simulink model "MDFM2"  (R2023a)
settings: Solver=FixedStepDiscrete  StartTime=0.0  StopTime=10.0  FixedStep=0.0001  RelTol=1e-3  EnableMultiTasking=on
undefined symbols (not defined in the file or in its folder): GLBCal_GLBCal_Kf_DCLinkOverVolErrThd_V, GLBCal_GLBCal_Kf_DCLinkUnderVolErrThd_V, KfMDFM_DCLinkOverVolWarnThd_V, KfMDFM_DCLinkUnderVolWarnThd_V, KfMDFM_OverVolPowerOutoutSetPoint_V, KfMDFM_OverVolPowerOutputFactor_NULL, KfMDFM_UnderVolPowerOutoutSetPoint_V, KfMDFM_UnderVolPowerOutputFactor_NULL, KuMDFM_DCLinkOVECntDownLimit_NULL, KuMDFM_DCLinkOVECntDownRate_NULL, KuMDFM_DCLinkOVECntUpLimit_NULL, KuMDFM_DCLinkOVECntUpRate_NULL, KuMDFM_DCLinkOVWCntDownLimit_NULL, KuMDFM_DCLinkOVWCntDownRate_NULL, KuMDFM_DCLinkOVWCntUpLimit_NULL, KuMDFM_DCLinkOVWCntUpRate_NULL, KuMDFM_DCLinkUVECntDownLimit_NULL, KuMDFM_DCLinkUVECntDownRate_NULL, KuMDFM_DCLinkUVECntUpLimit_NULL, KuMDFM_DCLinkUVECntUpRate_NULL, KuMDFM_DCLinkUVWCntDownLimit_NULL, KuMDFM_DCLinkUVWCntDownRate_NULL, KuMDFM_DCLinkUVWCntUpLimit_NULL, KuMDFM_DCLinkUVWCntUpRate_NULL, MDPM_MCUStatus, MDSM_MCUStatus
libraries: simulink x8, PMSM_Library x5
settings Model: DataDictionary=PMSM_Merge.sldd  EnableAccessToBaseWorkspace=off  Creator=yuliang  LastModifiedBy=洲
settings SolverCC: AlgebraicLoopSolver=TrustRegion
settings DataIOCC: LimitDataPoints=on  SaveFormat=StructureWithTime  ReturnWorkspaceOutputs=off
settings OptimizationCC: DefaultParameterBehavior=Inlined  DefaultUnderspecifiedDataType=single  EnhancedBackFolding=on  PassReuseOutputArgsAs=Individual arguments  ZeroExternalMemoryAtStartup=off  ZeroInternalMemoryAtStartup=off  OptimizeBlockOrder=speed  DifferentSizesBufferReuse=on  OptimizationCustomize=off  EfficientTunableParamExpr=on
settings DebuggingCC: ParameterTunabilityLossMsg=error  UnconnectedInputMsg=warning  UnconnectedOutputMsg=warning  UnconnectedLineMsg=warning  AllowSymbolicDim=off  SFUnexpectedBacktrackingDiag=warning  SFNoUnconditionalDefaultTransitionDiag=warning  SFExecutionAtInitializationDiag=none  ArithmeticOperatorsInVariantConditions=warning
settings HardwareCC: ProdBitPerPointer=32  ProdBitPerSizeT=32  ProdBitPerPtrDiffT=32  ProdLargestAtomicFloat=None  ProdWordSize=32  ProdHWDeviceType=Infineon->TriCore
settings ModelReferenceCC: EnableRefExpFcnMdlSchedulingChecks=on  ModelReferenceNumInstancesAllowed=Single  PropagateSignalLabelsOutOfModel=off
settings SFSimCC: SimUseLocalCustomCode=off  MATLABDynamicMemAlloc=off  CustomCodeUndefinedFunction=UseInterfaceOnly
settings RTWCC: Description=AUTOSAR  SystemTargetFile=autosar.tlc  GenCodeOnly=on  TemplateMakefile=ert_default_tmf  GenerateReport=on  RTWUseLocalCustomCode=off  IncludeHyperlinkInReport=on  LaunchReport=on  GenerateTraceInfo=on  GenerateTraceReport=on  GenerateTraceReportSl=on  GenerateTraceReportSf=on  GenerateTraceReportEml=on  DLArmComputeVersion=19.05
settings CodeAppCC: ForceParamTrailComments=on  IgnoreCustomStorageClasses=off  OperatorAnnotations=on  SimulinkDataObjDesc=on  SFDataObjDesc=on  InsertBlockDesc=on
settings STFCustomTargetCC: TargetLangStandard=C89/C90 (ANSI)  MultiwordLength=256  ParMdlRefBuildCompliant=on  CompOptLevelCompliant=on  ConcurrentExecutionCompliant=off  IncludeMdlTerminateFcn=off  CombineOutputUpdateFcns=on  SuppressErrorStatus=on  ERTCustomFileBanners=on  SupportNonFinite=off  SupportComplex=off  SupportContinuousTime=off  SupportNonInlinedSFcns=off  RemoveResetFunc=on  MATLABClassNameForMDSCustomization=Simulink.SoftwareTarget.ERTCustomization  AutosarCompliant=on  GRTInterface=off  LookupTableObjectStructAxisOrder=2,1,3,4,...  LUTObjectStructOrderEvenSpacing=Size,Table,Breakpoints  SystemTargetFile=autosar.tlc
settings ERTTargetCC: ConcurrentExecutionCompliant=off  IncludeMdlTerminateFcn=off  SuppressErrorStatus=on  SupportNonFinite=off  SupportComplex=off  ModelStepFunctionPrototypeControlCompliant=off  CPPClassGenCompliant=off  AutosarCompliant=on  LookupTableObjectStructAxisOrder=2,1,3,4,...  LUTObjectStructOrderEvenSpacing=Size,Table,Breakpoints  InlinedParameterPlacement=NonHierarchical  ERTCustomFileTemplate=example_file_process.tlc
settings ConfigComp: CovMetricSettings=dw  CovSaveCumulativeToWorkspaceVar=on  CovSaveSingleToWorkspaceVar=on  CovExternalEMLEnable=off

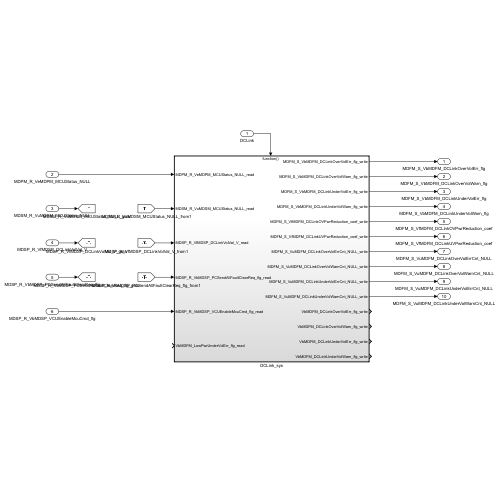
[thumbnail: Simulink's stored preview of the top-level diagram]
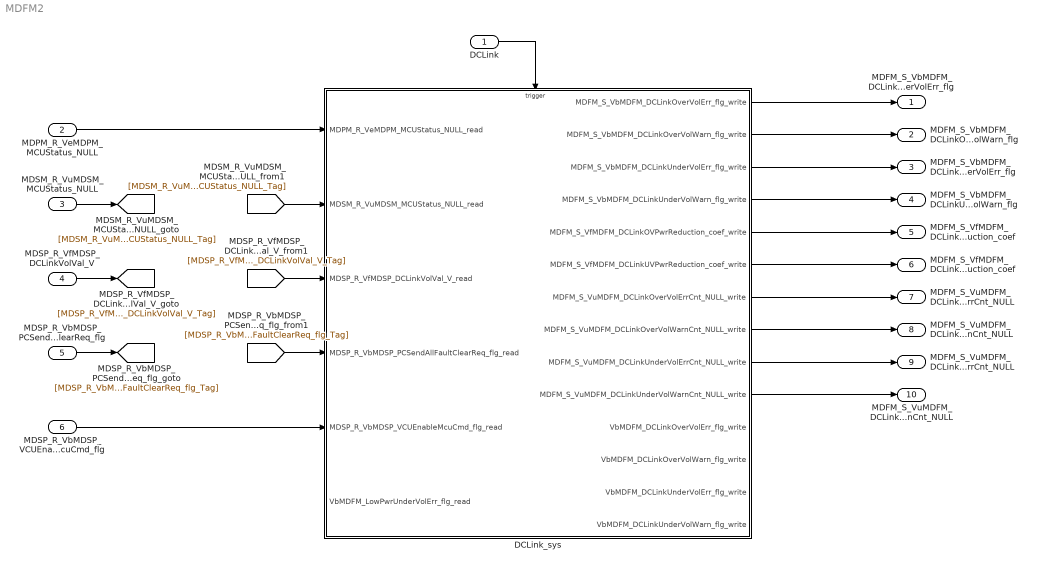
== system MDFM2 ==
  DCLink : Inport  SampleTime=0.005  OutputFunctionCall=on
  MDPM_R_VeMDPM_MCUStatus_NULL : Inport  Port=2  OutDataTypeStr=uint8  PortDimensions=1
  MDSM_R_VuMDSM_MCUStatus_NULL : Inport  Port=3  OutDataTypeStr=uint16  PortDimensions=1
  MDSP_R_VfMDSP_DCLinkVolVal_V : Inport  Port=4  OutDataTypeStr=single  PortDimensions=1
  MDSP_R_VbMDSP_PCSendAllFaultClearReq_flg : Inport  Port=5  OutDataTypeStr=boolean  PortDimensions=1
  MDSP_R_VbMDSP_VCUEnableMcuCmd_flg : Inport  Port=6  OutDataTypeStr=boolean  PortDimensions=1
  DCLink_sys : Subsystem
  MDFM_S_VbMDFM_DCLinkOverVolErr_flg : Outport  OutDataTypeStr=boolean  PortDimensions=1
  MDFM_S_VbMDFM_DCLinkOverVolWarn_flg : Outport  Port=2  OutDataTypeStr=boolean  PortDimensions=1
  MDFM_S_VbMDFM_DCLinkUnderVolErr_flg : Outport  Port=3  OutDataTypeStr=boolean  PortDimensions=1
  MDFM_S_VbMDFM_DCLinkUnderVolWarn_flg : Outport  Port=4  OutDataTypeStr=boolean  PortDimensions=1
  MDFM_S_VfMDFM_DCLinkOVPwrReduction_coef : Outport  Port=5  OutDataTypeStr=single  PortDimensions=1
  MDFM_S_VfMDFM_DCLinkUVPwrReduction_coef : Outport  Port=6  OutDataTypeStr=single  PortDimensions=1
  MDFM_S_VuMDFM_DCLinkOverVolErrCnt_NULL : Outport  Port=7  OutDataTypeStr=uint16  PortDimensions=1
  MDFM_S_VuMDFM_DCLinkOverVolWarnCnt_NULL : Outport  Port=8  OutDataTypeStr=uint16  PortDimensions=1
  MDFM_S_VuMDFM_DCLinkUnderVolErrCnt_NULL : Outport  Port=9  OutDataTypeStr=uint16  PortDimensions=1
  MDFM_S_VuMDFM_DCLinkUnderVolWarnCnt_NULL : Outport  Port=10  OutDataTypeStr=uint16  PortDimensions=1
  wires:
  DCLink/1 -> DCLink_sys/Trigger
  MDPM_R_VeMDPM_MCUStatus_NULL/1 -> DCLink_sys/1(MDPM_R_VeMDPM_MCUStatus_NULL_read)
  MDSM_R_VuMDSM_MCUStatus_NULL/1 -> [MDSM_R_VuMDSM_MCUStatus_NULL_Tag]
  [MDSM_R_VuMDSM_MCUStatus_NULL_Tag] -> DCLink_sys/2(MDSM_R_VuMDSM_MCUStatus_NULL_read)
  MDSP_R_VfMDSP_DCLinkVolVal_V/1 -> [MDSP_R_VfMDSP_DCLinkVolVal_V_Tag]
  [MDSP_R_VfMDSP_DCLinkVolVal_V_Tag] -> DCLink_sys/3(MDSP_R_VfMDSP_DCLinkVolVal_V_read)
  MDSP_R_VbMDSP_PCSendAllFaultClearReq_flg/1 -> [MDSP_R_VbMDSP_PCSendAllFaultClearReq_flg_Tag]
  [MDSP_R_VbMDSP_PCSendAllFaultClearReq_flg_Tag] -> DCLink_sys/4(MDSP_R_VbMDSP_PCSendAllFaultClearReq_flg_read)
  MDSP_R_VbMDSP_VCUEnableMcuCmd_flg/1 -> DCLink_sys/5(MDSP_R_VbMDSP_VCUEnableMcuCmd_flg_read)
  DCLink_sys/1(MDFM_S_VbMDFM_DCLinkOverVolErr_flg_write) -> MDFM_S_VbMDFM_DCLinkOverVolErr_flg/1
  DCLink_sys/2(MDFM_S_VbMDFM_DCLinkOverVolWarn_flg_write) -> MDFM_S_VbMDFM_DCLinkOverVolWarn_flg/1
  DCLink_sys/3(MDFM_S_VbMDFM_DCLinkUnderVolErr_flg_write) -> MDFM_S_VbMDFM_DCLinkUnderVolErr_flg/1
  DCLink_sys/4(MDFM_S_VbMDFM_DCLinkUnderVolWarn_flg_write) -> MDFM_S_VbMDFM_DCLinkUnderVolWarn_flg/1
  DCLink_sys/5(MDFM_S_VfMDFM_DCLinkOVPwrReduction_coef_write) -> MDFM_S_VfMDFM_DCLinkOVPwrReduction_coef/1
  DCLink_sys/6(MDFM_S_VfMDFM_DCLinkUVPwrReduction_coef_write) -> MDFM_S_VfMDFM_DCLinkUVPwrReduction_coef/1
  DCLink_sys/7(MDFM_S_VuMDFM_DCLinkOverVolErrCnt_NULL_write) -> MDFM_S_VuMDFM_DCLinkOverVolErrCnt_NULL/1
  DCLink_sys/8(MDFM_S_VuMDFM_DCLinkOverVolWarnCnt_NULL_write) -> MDFM_S_VuMDFM_DCLinkOverVolWarnCnt_NULL/1
  DCLink_sys/9(MDFM_S_VuMDFM_DCLinkUnderVolErrCnt_NULL_write) -> MDFM_S_VuMDFM_DCLinkUnderVolErrCnt_NULL/1
  DCLink_sys/10(MDFM_S_VuMDFM_DCLinkUnderVolWarnCnt_NULL_write) -> MDFM_S_VuMDFM_DCLinkUnderVolWarnCnt_NULL/1

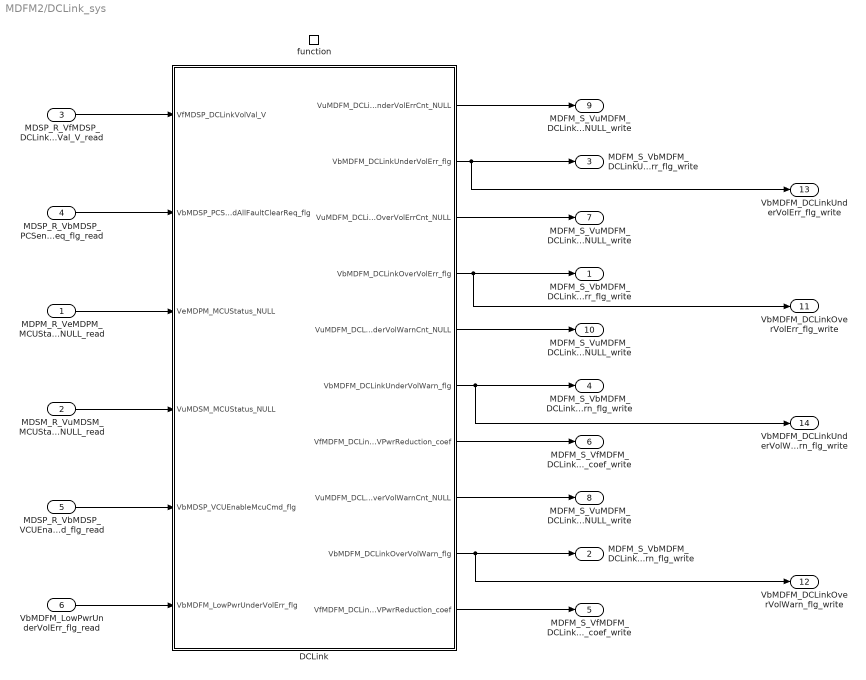
== system MDFM2/DCLink_sys ==
  MDPM_R_VeMDPM_MCUStatus_NULL_read : Inport
  MDSM_R_VuMDSM_MCUStatus_NULL_read : Inport  Port=2
  MDSP_R_VfMDSP_DCLinkVolVal_V_read : Inport  Port=3
  MDSP_R_VbMDSP_PCSendAllFaultClearReq_flg_read : Inport  Port=4
  MDSP_R_VbMDSP_VCUEnableMcuCmd_flg_read : Inport  Port=5
  VbMDFM_LowPwrUnderVolErr_flg_read : Inport  Port=6
  function : TriggerPort  TriggerType=function-call  VariantControl=Variant  SampleTimeType=periodic  SampleTime=-1
  DCLink : Subsystem
  MDFM_S_VbMDFM_DCLinkOverVolErr_flg_write : Outport
  MDFM_S_VbMDFM_DCLinkOverVolWarn_flg_write : Outport  Port=2
  MDFM_S_VbMDFM_DCLinkUnderVolErr_flg_write : Outport  Port=3
  MDFM_S_VbMDFM_DCLinkUnderVolWarn_flg_write : Outport  Port=4
  MDFM_S_VfMDFM_DCLinkOVPwrReduction_coef_write : Outport  Port=5
  MDFM_S_VfMDFM_DCLinkUVPwrReduction_coef_write : Outport  Port=6
  MDFM_S_VuMDFM_DCLinkOverVolErrCnt_NULL_write : Outport  Port=7
  MDFM_S_VuMDFM_DCLinkOverVolWarnCnt_NULL_write : Outport  Port=8
  MDFM_S_VuMDFM_DCLinkUnderVolErrCnt_NULL_write : Outport  Port=9
  MDFM_S_VuMDFM_DCLinkUnderVolWarnCnt_NULL_write : Outport  Port=10
  VbMDFM_DCLinkOverVolErr_flg_write : Outport  Port=11  OutDataTypeStr=boolean  PortDimensions=1
  VbMDFM_DCLinkOverVolWarn_flg_write : Outport  Port=12  OutDataTypeStr=boolean  PortDimensions=1
  VbMDFM_DCLinkUnderVolErr_flg_write : Outport  Port=13  OutDataTypeStr=boolean  PortDimensions=1
  VbMDFM_DCLinkUnderVolWarn_flg_write : Outport  Port=14  OutDataTypeStr=boolean  PortDimensions=1
  wires:
  MDPM_R_VeMDPM_MCUStatus_NULL_read/1 -> DCLink/3(VeMDPM_MCUStatus_NULL)
  MDSM_R_VuMDSM_MCUStatus_NULL_read/1 -> DCLink/4(VuMDSM_MCUStatus_NULL)
  MDSP_R_VfMDSP_DCLinkVolVal_V_read/1 -> DCLink/1(VfMDSP_DCLinkVolVal_V)
  MDSP_R_VbMDSP_PCSendAllFaultClearReq_flg_read/1 -> DCLink/2(VbMDSP_PCSendAllFaultClearReq_flg)
  MDSP_R_VbMDSP_VCUEnableMcuCmd_flg_read/1 -> DCLink/5(VbMDSP_VCUEnableMcuCmd_flg)
  VbMDFM_LowPwrUnderVolErr_flg_read/1 -> DCLink/6(VbMDFM_LowPwrUnderVolErr_flg)
  DCLink/9(VbMDFM_DCLinkOverVolWarn_flg) -> VbMDFM_DCLinkOverVolWarn_flg_write/1, MDFM_S_VbMDFM_DCLinkOverVolWarn_flg_write/1
  DCLink/10(VfMDFM_DCLinkOVPwrReduction_coef) -> MDFM_S_VfMDFM_DCLinkOVPwrReduction_coef_write/1
  DCLink/7(VfMDFM_DCLinkUVPwrReduction_coef) -> MDFM_S_VfMDFM_DCLinkUVPwrReduction_coef_write/1
  DCLink/3(VuMDFM_DCLinkOverVolErrCnt_NULL) -> MDFM_S_VuMDFM_DCLinkOverVolErrCnt_NULL_write/1
  DCLink/1(VuMDFM_DCLinkUnderVolErrCnt_NULL) -> MDFM_S_VuMDFM_DCLinkUnderVolErrCnt_NULL_write/1
  DCLink/5(VuMDFM_DCLinkUnderVolWarnCnt_NULL) -> MDFM_S_VuMDFM_DCLinkUnderVolWarnCnt_NULL_write/1
  DCLink/4(VbMDFM_DCLinkOverVolErr_flg) -> VbMDFM_DCLinkOverVolErr_flg_write/1, MDFM_S_VbMDFM_DCLinkOverVolErr_flg_write/1
  DCLink/8(VuMDFM_DCLinkOverVolWarnCnt_NULL) -> MDFM_S_VuMDFM_DCLinkOverVolWarnCnt_NULL_write/1
  DCLink/2(VbMDFM_DCLinkUnderVolErr_flg) -> VbMDFM_DCLinkUnderVolErr_flg_write/1, MDFM_S_VbMDFM_DCLinkUnderVolErr_flg_write/1
  DCLink/6(VbMDFM_DCLinkUnderVolWarn_flg) -> VbMDFM_DCLinkUnderVolWarn_flg_write/1, MDFM_S_VbMDFM_DCLinkUnderVolWarn_flg_write/1

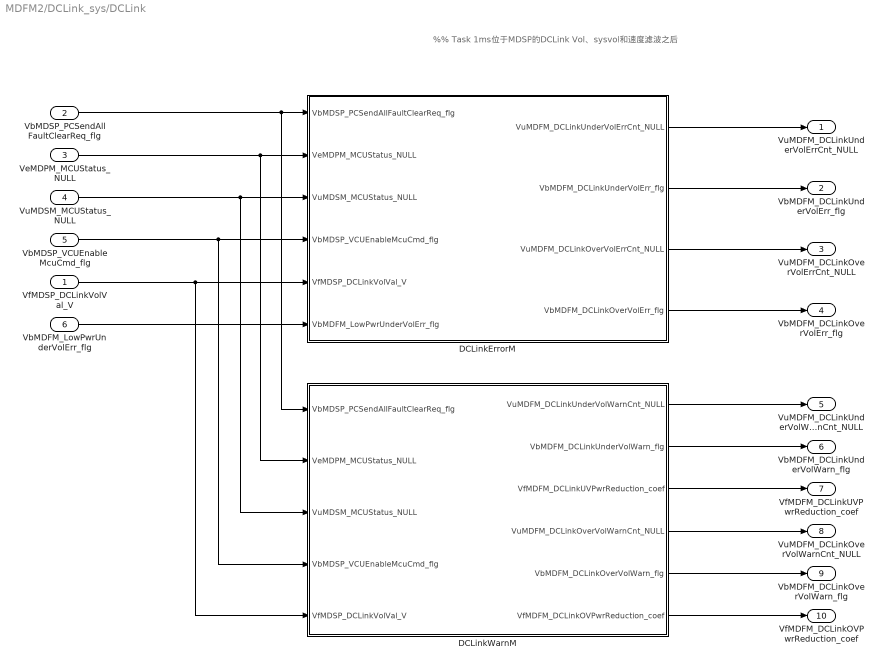
== system MDFM2/DCLink_sys/DCLink ==
  note: %% Task 1ms位于MDSP的DCLink Vol、sysvol和速度滤波之后
  VfMDSP_DCLinkVolVal_V : Inport
  VbMDSP_PCSendAllFaultClearReq_flg : Inport  Port=2
  VeMDPM_MCUStatus_NULL : Inport  Port=3
  VuMDSM_MCUStatus_NULL : Inport  Port=4
  VbMDSP_VCUEnableMcuCmd_flg : Inport  Port=5
  VbMDFM_LowPwrUnderVolErr_flg : Inport  Port=6
  DCLinkErrorM : Subsystem  TreatAsAtomicUnit=on  RTWFcnName=MDFM_DCLinkErrorM  RTWFileName=MDFM
      settings: RTWSystemCode=Nonreusable function  RTWFcnNameOpts=User specified
  DCLinkWarnM : Subsystem  TreatAsAtomicUnit=on  RTWFcnName=MDFM_DCLinkWarnM  RTWFileName=MDFM
      settings: RTWSystemCode=Nonreusable function  RTWFcnNameOpts=User specified
  VuMDFM_DCLinkUnderVolErrCnt_NULL : Outport
  VbMDFM_DCLinkUnderVolErr_flg : Outport  Port=2
  VuMDFM_DCLinkOverVolErrCnt_NULL : Outport  Port=3
  VbMDFM_DCLinkOverVolErr_flg : Outport  Port=4
  VuMDFM_DCLinkUnderVolWarnCnt_NULL : Outport  Port=5
  VbMDFM_DCLinkUnderVolWarn_flg : Outport  Port=6
  VfMDFM_DCLinkUVPwrReduction_coef : Outport  Port=7
  VuMDFM_DCLinkOverVolWarnCnt_NULL : Outport  Port=8
  VbMDFM_DCLinkOverVolWarn_flg : Outport  Port=9
  VfMDFM_DCLinkOVPwrReduction_coef : Outport  Port=10
  wires:
  DCLinkErrorM/4(VbMDFM_DCLinkOverVolErr_flg) -> VbMDFM_DCLinkOverVolErr_flg/1
  DCLinkErrorM/3(VuMDFM_DCLinkOverVolErrCnt_NULL) -> VuMDFM_DCLinkOverVolErrCnt_NULL/1
  DCLinkErrorM/2(VbMDFM_DCLinkUnderVolErr_flg) -> VbMDFM_DCLinkUnderVolErr_flg/1
  DCLinkErrorM/1(VuMDFM_DCLinkUnderVolErrCnt_NULL) -> VuMDFM_DCLinkUnderVolErrCnt_NULL/1
  DCLinkWarnM/1(VuMDFM_DCLinkUnderVolWarnCnt_NULL) -> VuMDFM_DCLinkUnderVolWarnCnt_NULL/1
  DCLinkWarnM/2(VbMDFM_DCLinkUnderVolWarn_flg) -> VbMDFM_DCLinkUnderVolWarn_flg/1
  DCLinkWarnM/3(VfMDFM_DCLinkUVPwrReduction_coef) -> VfMDFM_DCLinkUVPwrReduction_coef/1
  DCLinkWarnM/4(VuMDFM_DCLinkOverVolWarnCnt_NULL) -> VuMDFM_DCLinkOverVolWarnCnt_NULL/1
  DCLinkWarnM/5(VbMDFM_DCLinkOverVolWarn_flg) -> VbMDFM_DCLinkOverVolWarn_flg/1
  DCLinkWarnM/6(VfMDFM_DCLinkOVPwrReduction_coef) -> VfMDFM_DCLinkOVPwrReduction_coef/1
  VbMDSP_PCSendAllFaultClearReq_flg/1 -> DCLinkWarnM/1(VbMDSP_PCSendAllFaultClearReq_flg), DCLinkErrorM/1(VbMDSP_PCSendAllFaultClearReq_flg)
  VeMDPM_MCUStatus_NULL/1 -> DCLinkWarnM/2(VeMDPM_MCUStatus_NULL), DCLinkErrorM/2(VeMDPM_MCUStatus_NULL)
  VuMDSM_MCUStatus_NULL/1 -> DCLinkWarnM/3(VuMDSM_MCUStatus_NULL), DCLinkErrorM/3(VuMDSM_MCUStatus_NULL)
  VbMDSP_VCUEnableMcuCmd_flg/1 -> DCLinkWarnM/4(VbMDSP_VCUEnableMcuCmd_flg), DCLinkErrorM/4(VbMDSP_VCUEnableMcuCmd_flg)
  VfMDSP_DCLinkVolVal_V/1 -> DCLinkWarnM/5(VfMDSP_DCLinkVolVal_V), DCLinkErrorM/5(VfMDSP_DCLinkVolVal_V)
  VbMDFM_LowPwrUnderVolErr_flg/1 -> DCLinkErrorM/6(VbMDFM_LowPwrUnderVolErr_flg)

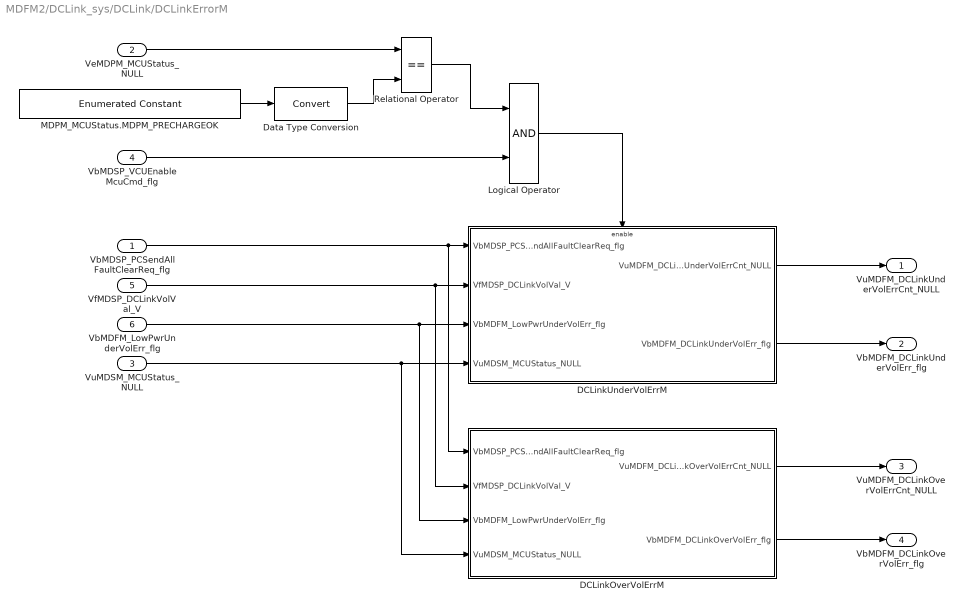
== system MDFM2/DCLink_sys/DCLink/DCLinkErrorM ==
  VbMDSP_PCSendAllFaultClearReq_flg : Inport
  VeMDPM_MCUStatus_NULL : Inport  Port=2
  VuMDSM_MCUStatus_NULL : Inport  Port=3
  VbMDSP_VCUEnableMcuCmd_flg : Inport  Port=4
  VfMDSP_DCLinkVolVal_V : Inport  Port=5
  VbMDFM_LowPwrUnderVolErr_flg : Inport  Port=6
  DCLinkOverVolErrM : Subsystem  TreatAsAtomicUnit=on  RTWFileName=MDFM
      settings: RTWSystemCode=Nonreusable function  RTWFcnNameOpts=Use subsystem name  FunctionInterfaceSpec=Allow arguments (Optimized)
  DCLinkUnderVolErrM : Subsystem  TreatAsAtomicUnit=on
      settings: RTWSystemCode=Nonreusable function  RTWFcnNameOpts=Use subsystem name
  Data Type Conversion : DataTypeConversion  SaturateOnIntegerOverflow=off  RndMeth=Floor
  Logical Operator : Logic  AllPortsSameDT=off  OutDataTypeStr=boolean
  MDPM_MCUStatus.MDPM_PRECHARGEOK : simulink/Sources/Enumerated Constant  OutDataTypeStr=Enum: MDPM_MCUStatus  Value=MDPM_MCUStatus.MDPM_PRECHARGEOK  SampleTime=-1
  Relational Operator : RelationalOperator  Operator===  OutDataTypeStr=boolean  InputSameDT=off
  VuMDFM_DCLinkUnderVolErrCnt_NULL : Outport
  VbMDFM_DCLinkUnderVolErr_flg : Outport  Port=2
  VuMDFM_DCLinkOverVolErrCnt_NULL : Outport  Port=3
  VbMDFM_DCLinkOverVolErr_flg : Outport  Port=4
  wires:
  VeMDPM_MCUStatus_NULL/1 -> Relational Operator/1
  MDPM_MCUStatus.MDPM_PRECHARGEOK/1 -> Data Type Conversion/1
  Data Type Conversion/1 -> Relational Operator/2
  Relational Operator/1 -> Logical Operator/1
  Logical Operator/1 -> DCLinkUnderVolErrM/Enable
  VbMDSP_VCUEnableMcuCmd_flg/1 -> Logical Operator/2
  DCLinkUnderVolErrM/2(VbMDFM_DCLinkUnderVolErr_flg) -> VbMDFM_DCLinkUnderVolErr_flg/1
  DCLinkUnderVolErrM/1(VuMDFM_DCLinkUnderVolErrCnt_NULL) -> VuMDFM_DCLinkUnderVolErrCnt_NULL/1
  DCLinkOverVolErrM/2(VbMDFM_DCLinkOverVolErr_flg) -> VbMDFM_DCLinkOverVolErr_flg/1
  DCLinkOverVolErrM/1(VuMDFM_DCLinkOverVolErrCnt_NULL) -> VuMDFM_DCLinkOverVolErrCnt_NULL/1
  VbMDFM_LowPwrUnderVolErr_flg/1 -> DCLinkOverVolErrM/3(VbMDFM_LowPwrUnderVolErr_flg), DCLinkUnderVolErrM/3(VbMDFM_LowPwrUnderVolErr_flg)
  VuMDSM_MCUStatus_NULL/1 -> DCLinkOverVolErrM/4(VuMDSM_MCUStatus_NULL), DCLinkUnderVolErrM/4(VuMDSM_MCUStatus_NULL)
  VfMDSP_DCLinkVolVal_V/1 -> DCLinkOverVolErrM/2(VfMDSP_DCLinkVolVal_V), DCLinkUnderVolErrM/2(VfMDSP_DCLinkVolVal_V)
  VbMDSP_PCSendAllFaultClearReq_flg/1 -> DCLinkOverVolErrM/1(VbMDSP_PCSendAllFaultClearReq_flg), DCLinkUnderVolErrM/1(VbMDSP_PCSendAllFaultClearReq_flg)

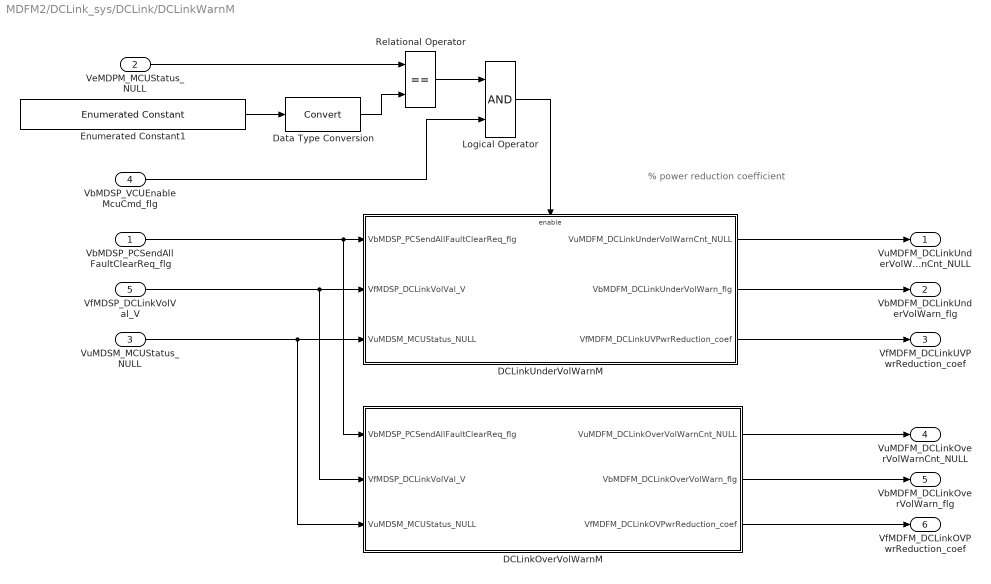
== system MDFM2/DCLink_sys/DCLink/DCLinkWarnM ==
  note: % power reduction coefficient
  VbMDSP_PCSendAllFaultClearReq_flg : Inport
  VeMDPM_MCUStatus_NULL : Inport  Port=2
  VuMDSM_MCUStatus_NULL : Inport  Port=3
  VbMDSP_VCUEnableMcuCmd_flg : Inport  Port=4
  VfMDSP_DCLinkVolVal_V : Inport  Port=5
  DCLinkOverVolWarnM : Subsystem  TreatAsAtomicUnit=on
      settings: RTWSystemCode=Nonreusable function  RTWFcnNameOpts=Use subsystem name
  DCLinkUnderVolWarnM : Subsystem  TreatAsAtomicUnit=on
      settings: RTWSystemCode=Nonreusable function  RTWFcnNameOpts=Use subsystem name
  Data Type Conversion : DataTypeConversion  SaturateOnIntegerOverflow=off  RndMeth=Floor
  Enumerated Constant1 : simulink/Sources/Enumerated Constant  OutDataTypeStr=Enum: MDPM_MCUStatus  Value=MDPM_MCUStatus.MDPM_PRECHARGEOK  SampleTime=-1
  Logical Operator : Logic  AllPortsSameDT=off  OutDataTypeStr=boolean
  Relational Operator : RelationalOperator  Operator===  OutDataTypeStr=boolean  InputSameDT=off
  VuMDFM_DCLinkUnderVolWarnCnt_NULL : Outport
  VbMDFM_DCLinkUnderVolWarn_flg : Outport  Port=2
  VfMDFM_DCLinkUVPwrReduction_coef : Outport  Port=3
  VuMDFM_DCLinkOverVolWarnCnt_NULL : Outport  Port=4
  VbMDFM_DCLinkOverVolWarn_flg : Outport  Port=5
  VfMDFM_DCLinkOVPwrReduction_coef : Outport  Port=6
  wires:
  VeMDPM_MCUStatus_NULL/1 -> Relational Operator/1
  Enumerated Constant1/1 -> Data Type Conversion/1
  Data Type Conversion/1 -> Relational Operator/2
  Logical Operator/1 -> DCLinkUnderVolWarnM/Enable
  Relational Operator/1 -> Logical Operator/1
  VbMDSP_VCUEnableMcuCmd_flg/1 -> Logical Operator/2
  VbMDSP_PCSendAllFaultClearReq_flg/1 -> DCLinkOverVolWarnM/1(VbMDSP_PCSendAllFaultClearReq_flg), DCLinkUnderVolWarnM/1(VbMDSP_PCSendAllFaultClearReq_flg)
  VfMDSP_DCLinkVolVal_V/1 -> DCLinkOverVolWarnM/2(VfMDSP_DCLinkVolVal_V), DCLinkUnderVolWarnM/2(VfMDSP_DCLinkVolVal_V)
  VuMDSM_MCUStatus_NULL/1 -> DCLinkOverVolWarnM/3(VuMDSM_MCUStatus_NULL), DCLinkUnderVolWarnM/3(VuMDSM_MCUStatus_NULL)
  DCLinkUnderVolWarnM/1(VuMDFM_DCLinkUnderVolWarnCnt_NULL) -> VuMDFM_DCLinkUnderVolWarnCnt_NULL/1
  DCLinkUnderVolWarnM/2(VbMDFM_DCLinkUnderVolWarn_flg) -> VbMDFM_DCLinkUnderVolWarn_flg/1
  DCLinkUnderVolWarnM/3(VfMDFM_DCLinkUVPwrReduction_coef) -> VfMDFM_DCLinkUVPwrReduction_coef/1
  DCLinkOverVolWarnM/2(VbMDFM_DCLinkOverVolWarn_flg) -> VbMDFM_DCLinkOverVolWarn_flg/1
  DCLinkOverVolWarnM/1(VuMDFM_DCLinkOverVolWarnCnt_NULL) -> VuMDFM_DCLinkOverVolWarnCnt_NULL/1
  DCLinkOverVolWarnM/3(VfMDFM_DCLinkOVPwrReduction_coef) -> VfMDFM_DCLinkOVPwrReduction_coef/1

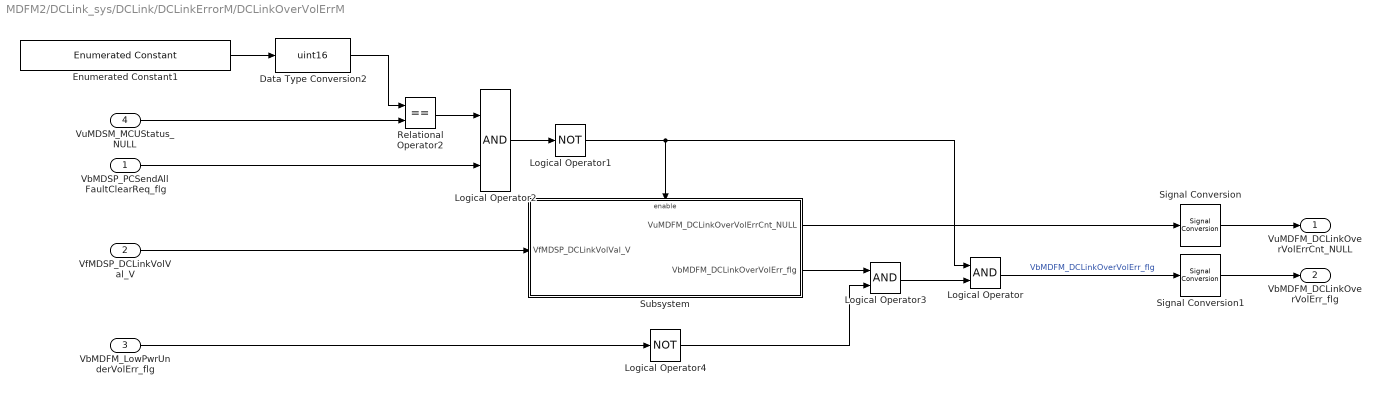
== system MDFM2/DCLink_sys/DCLink/DCLinkErrorM/DCLinkOverVolErrM ==
  VbMDSP_PCSendAllFaultClearReq_flg : Inport
  VfMDSP_DCLinkVolVal_V : Inport  Port=2
  VbMDFM_LowPwrUnderVolErr_flg : Inport  Port=3
  VuMDSM_MCUStatus_NULL : Inport  Port=4
  Data Type Conversion2 : DataTypeConversion  OutDataTypeStr=uint16  SaturateOnIntegerOverflow=off  RndMeth=Floor
  Enumerated Constant1 : simulink/Sources/Enumerated Constant  OutDataTypeStr=Enum: MDSM_MCUStatus  Value=MDSM_MCUStatus.MDSM_FailureHandle  SampleTime=inf
  Logical Operator : Logic  AllPortsSameDT=off  OutDataTypeStr=boolean
  Logical Operator1 : Logic  Operator=NOT  AllPortsSameDT=off  OutDataTypeStr=boolean
  Logical Operator2 : Logic  AllPortsSameDT=off  OutDataTypeStr=boolean
  Logical Operator3 : Logic  AllPortsSameDT=off  OutDataTypeStr=boolean
  Logical Operator4 : Logic  Operator=NOT  AllPortsSameDT=off  OutDataTypeStr=boolean
  Relational Operator2 : RelationalOperator  Operator===  OutDataTypeStr=boolean  InputSameDT=off
  Signal Conversion : SignalConversion  OverrideOpt=off
  Signal Conversion1 : SignalConversion  OverrideOpt=off
  Subsystem : Subsystem
  VuMDFM_DCLinkOverVolErrCnt_NULL : Outport
  VbMDFM_DCLinkOverVolErr_flg : Outport  Port=2
  wires:
  Subsystem/1(VuMDFM_DCLinkOverVolErrCnt_NULL) -> Signal Conversion/1
  Logical Operator/1 -> Signal Conversion1/1  "VbMDFM_DCLinkOverVolErr_flg"
  VbMDSP_PCSendAllFaultClearReq_flg/1 -> Logical Operator2/2
  Enumerated Constant1/1 -> Data Type Conversion2/1
  Data Type Conversion2/1 -> Relational Operator2/1
  Relational Operator2/1 -> Logical Operator2/1
  VuMDSM_MCUStatus_NULL/1 -> Relational Operator2/2
  Logical Operator2/1 -> Logical Operator1/1
  Logical Operator1/1 -> Logical Operator/1, Subsystem/Enable
  Subsystem/2(VbMDFM_DCLinkOverVolErr_flg) -> Logical Operator3/1
  VfMDSP_DCLinkVolVal_V/1 -> Subsystem/1(VfMDSP_DCLinkVolVal_V)
  Logical Operator4/1 -> Logical Operator3/2
  VbMDFM_LowPwrUnderVolErr_flg/1 -> Logical Operator4/1
  Logical Operator3/1 -> Logical Operator/2
  Signal Conversion/1 -> VuMDFM_DCLinkOverVolErrCnt_NULL/1
  Signal Conversion1/1 -> VbMDFM_DCLinkOverVolErr_flg/1

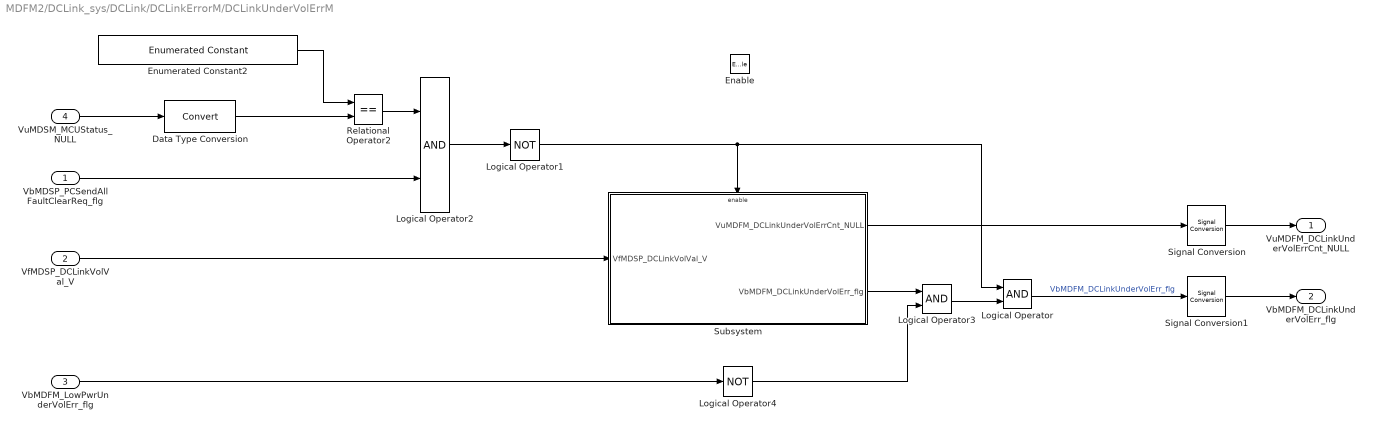
== system MDFM2/DCLink_sys/DCLink/DCLinkErrorM/DCLinkUnderVolErrM ==
  VbMDSP_PCSendAllFaultClearReq_flg : Inport
  VfMDSP_DCLinkVolVal_V : Inport  Port=2
  VbMDFM_LowPwrUnderVolErr_flg : Inport  Port=3
  VuMDSM_MCUStatus_NULL : Inport  Port=4
  Enable : EnablePort
  Data Type Conversion : DataTypeConversion  SaturateOnIntegerOverflow=off  RndMeth=Floor
  Enumerated Constant2 : simulink/Sources/Enumerated Constant  OutDataTypeStr=Enum: MDSM_MCUStatus  Value=MDSM_MCUStatus.MDSM_FailureHandle  SampleTime=inf
  Logical Operator : Logic  AllPortsSameDT=off  OutDataTypeStr=boolean
  Logical Operator1 : Logic  Operator=NOT  AllPortsSameDT=off  OutDataTypeStr=boolean
  Logical Operator2 : Logic  AllPortsSameDT=off  OutDataTypeStr=boolean
  Logical Operator3 : Logic  AllPortsSameDT=off  OutDataTypeStr=boolean
  Logical Operator4 : Logic  Operator=NOT  AllPortsSameDT=off  OutDataTypeStr=boolean
  Relational Operator2 : RelationalOperator  Operator===  OutDataTypeStr=boolean  InputSameDT=off
  Signal Conversion : SignalConversion  OverrideOpt=off
  Signal Conversion1 : SignalConversion  OverrideOpt=off
  Subsystem : Subsystem
  VuMDFM_DCLinkUnderVolErrCnt_NULL : Outport
  VbMDFM_DCLinkUnderVolErr_flg : Outport  Port=2
  wires:
  Subsystem/1(VuMDFM_DCLinkUnderVolErrCnt_NULL) -> Signal Conversion/1
  VbMDSP_PCSendAllFaultClearReq_flg/1 -> Logical Operator2/2
  Logical Operator/1 -> Signal Conversion1/1  "VbMDFM_DCLinkUnderVolErr_flg"
  Subsystem/2(VbMDFM_DCLinkUnderVolErr_flg) -> Logical Operator3/1
  Logical Operator1/1 -> Logical Operator/1, Subsystem/Enable
  Enumerated Constant2/1 -> Relational Operator2/1
  Relational Operator2/1 -> Logical Operator2/1
  VuMDSM_MCUStatus_NULL/1 -> Data Type Conversion/1
  Logical Operator2/1 -> Logical Operator1/1
  Data Type Conversion/1 -> Relational Operator2/2
  VfMDSP_DCLinkVolVal_V/1 -> Subsystem/1(VfMDSP_DCLinkVolVal_V)
  Logical Operator3/1 -> Logical Operator/2
  VbMDFM_LowPwrUnderVolErr_flg/1 -> Logical Operator4/1
  Logical Operator4/1 -> Logical Operator3/2
  Signal Conversion/1 -> VuMDFM_DCLinkUnderVolErrCnt_NULL/1
  Signal Conversion1/1 -> VbMDFM_DCLinkUnderVolErr_flg/1

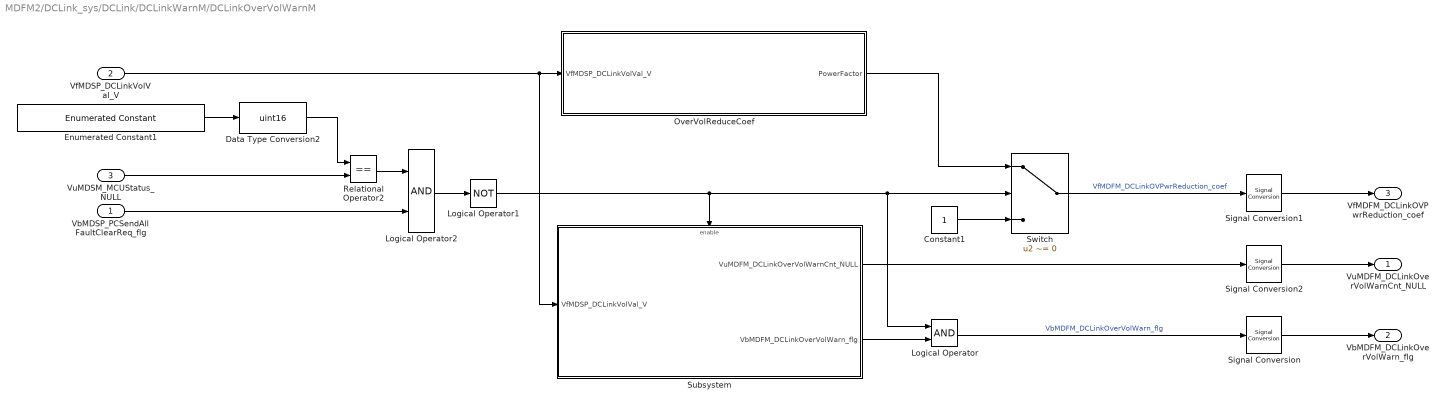
== system MDFM2/DCLink_sys/DCLink/DCLinkWarnM/DCLinkOverVolWarnM ==
  VbMDSP_PCSendAllFaultClearReq_flg : Inport
  VfMDSP_DCLinkVolVal_V : Inport  Port=2
  VuMDSM_MCUStatus_NULL : Inport  Port=3
  Constant1 : Constant  OutDataTypeStr=single
  Data Type Conversion2 : DataTypeConversion  OutDataTypeStr=uint16  SaturateOnIntegerOverflow=off  RndMeth=Floor
  Enumerated Constant1 : simulink/Sources/Enumerated Constant  OutDataTypeStr=Enum: MDSM_MCUStatus  Value=MDSM_MCUStatus.MDSM_FailureHandle  SampleTime=inf
  Logical Operator : Logic  AllPortsSameDT=off  OutDataTypeStr=boolean
  Logical Operator1 : Logic  Operator=NOT  AllPortsSameDT=off  OutDataTypeStr=boolean
  Logical Operator2 : Logic  AllPortsSameDT=off  OutDataTypeStr=boolean
  OverVolReduceCoef : Subsystem  TreatAsAtomicUnit=on
  Relational Operator2 : RelationalOperator  Operator===  OutDataTypeStr=boolean  InputSameDT=off
  Signal Conversion : SignalConversion  OverrideOpt=off
  Signal Conversion1 : SignalConversion  OverrideOpt=off
  Signal Conversion2 : SignalConversion  OverrideOpt=off
  Subsystem : Subsystem
  Switch : Switch  Criteria=u2 ~= 0  OutDataTypeStr=single  SaturateOnIntegerOverflow=off  InputSameDT=off
  VuMDFM_DCLinkOverVolWarnCnt_NULL : Outport
  VbMDFM_DCLinkOverVolWarn_flg : Outport  Port=2
  VfMDFM_DCLinkOVPwrReduction_coef : Outport  Port=3
  wires:
  Subsystem/1(VuMDFM_DCLinkOverVolWarnCnt_NULL) -> Signal Conversion2/1
  Logical Operator/1 -> Signal Conversion/1  "VbMDFM_DCLinkOverVolWarn_flg"
  Switch/1 -> Signal Conversion1/1  "VfMDFM_DCLinkOVPwrReduction_coef"
  Enumerated Constant1/1 -> Data Type Conversion2/1
  Data Type Conversion2/1 -> Relational Operator2/1
  Relational Operator2/1 -> Logical Operator2/1
  VuMDSM_MCUStatus_NULL/1 -> Relational Operator2/2
  Logical Operator2/1 -> Logical Operator1/1
  VbMDSP_PCSendAllFaultClearReq_flg/1 -> Logical Operator2/2
  Logical Operator1/1 -> Switch/2, Logical Operator/1, Subsystem/Enable
  Subsystem/2(VbMDFM_DCLinkOverVolWarn_flg) -> Logical Operator/2
  Constant1/1 -> Switch/3
  OverVolReduceCoef/1(PowerFactor) -> Switch/1
  VfMDSP_DCLinkVolVal_V/1 -> OverVolReduceCoef/1(VfMDSP_DCLinkVolVal_V), Subsystem/1(VfMDSP_DCLinkVolVal_V)
  Signal Conversion/1 -> VbMDFM_DCLinkOverVolWarn_flg/1
  Signal Conversion1/1 -> VfMDFM_DCLinkOVPwrReduction_coef/1
  Signal Conversion2/1 -> VuMDFM_DCLinkOverVolWarnCnt_NULL/1

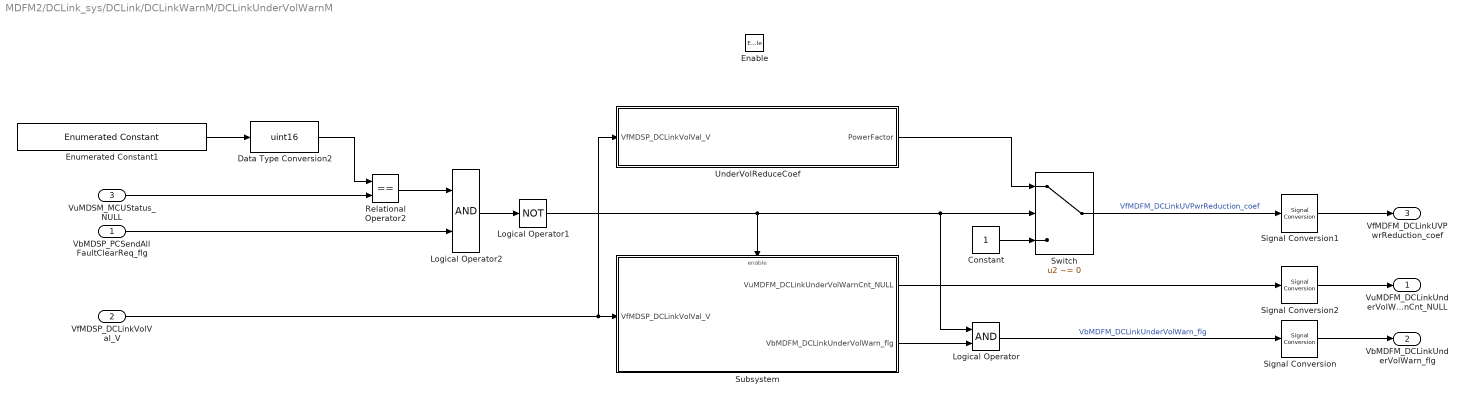
== system MDFM2/DCLink_sys/DCLink/DCLinkWarnM/DCLinkUnderVolWarnM ==
  VbMDSP_PCSendAllFaultClearReq_flg : Inport
  VfMDSP_DCLinkVolVal_V : Inport  Port=2
  VuMDSM_MCUStatus_NULL : Inport  Port=3
  Enable : EnablePort
  Constant : Constant  OutDataTypeStr=single
  Data Type Conversion2 : DataTypeConversion  OutDataTypeStr=uint16  SaturateOnIntegerOverflow=off  RndMeth=Floor
  Enumerated Constant1 : simulink/Sources/Enumerated Constant  OutDataTypeStr=Enum: MDSM_MCUStatus  Value=MDSM_MCUStatus.MDSM_FailureHandle  SampleTime=inf
  Logical Operator : Logic  AllPortsSameDT=off  OutDataTypeStr=boolean
  Logical Operator1 : Logic  Operator=NOT  AllPortsSameDT=off  OutDataTypeStr=boolean
  Logical Operator2 : Logic  AllPortsSameDT=off  OutDataTypeStr=boolean
  Relational Operator2 : RelationalOperator  Operator===  OutDataTypeStr=boolean  InputSameDT=off
  Signal Conversion : SignalConversion  OverrideOpt=off
  Signal Conversion1 : SignalConversion  OverrideOpt=off
  Signal Conversion2 : SignalConversion  OverrideOpt=off
  Subsystem : Subsystem
  Switch : Switch  Criteria=u2 ~= 0  SaturateOnIntegerOverflow=off  InputSameDT=off
  UnderVolReduceCoef : Subsystem  TreatAsAtomicUnit=on
  VuMDFM_DCLinkUnderVolWarnCnt_NULL : Outport
  VbMDFM_DCLinkUnderVolWarn_flg : Outport  Port=2
  VfMDFM_DCLinkUVPwrReduction_coef : Outport  Port=3
  wires:
  Subsystem/1(VuMDFM_DCLinkUnderVolWarnCnt_NULL) -> Signal Conversion2/1
  Logical Operator/1 -> Signal Conversion/1  "VbMDFM_DCLinkUnderVolWarn_flg"
  Switch/1 -> Signal Conversion1/1  "VfMDFM_DCLinkUVPwrReduction_coef"
  VbMDSP_PCSendAllFaultClearReq_flg/1 -> Logical Operator2/2
  Enumerated Constant1/1 -> Data Type Conversion2/1
  Data Type Conversion2/1 -> Relational Operator2/1
  Relational Operator2/1 -> Logical Operator2/1
  VuMDSM_MCUStatus_NULL/1 -> Relational Operator2/2
  Logical Operator2/1 -> Logical Operator1/1
  Logical Operator1/1 -> Switch/2, Logical Operator/1, Subsystem/Enable
  Subsystem/2(VbMDFM_DCLinkUnderVolWarn_flg) -> Logical Operator/2
  Constant/1 -> Switch/3
  UnderVolReduceCoef/1(PowerFactor) -> Switch/1
  VfMDSP_DCLinkVolVal_V/1 -> UnderVolReduceCoef/1(VfMDSP_DCLinkVolVal_V), Subsystem/1(VfMDSP_DCLinkVolVal_V)
  Signal Conversion/1 -> VbMDFM_DCLinkUnderVolWarn_flg/1
  Signal Conversion1/1 -> VfMDFM_DCLinkUVPwrReduction_coef/1
  Signal Conversion2/1 -> VuMDFM_DCLinkUnderVolWarnCnt_NULL/1

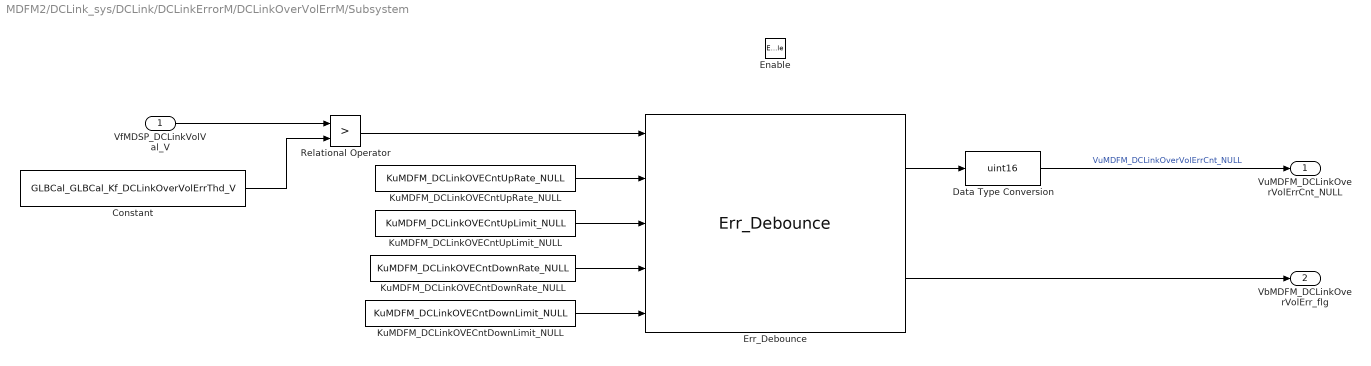
== system MDFM2/DCLink_sys/DCLink/DCLinkErrorM/DCLinkOverVolErrM/Subsystem ==
  VfMDSP_DCLinkVolVal_V : Inport
  Enable : EnablePort  StatesWhenEnabling=reset
      settings: AttributesFormatString=%<StatesWhenEnabling>
  Constant : Constant  Value=GLBCal_GLBCal_Kf_DCLinkOverVolErrThd_V
  Data Type Conversion : DataTypeConversion  OutDataTypeStr=uint16  SaturateOnIntegerOverflow=off  RndMeth=Floor
  Err_Debounce : PMSM_Library/Err_Debounce  SystemSampleTime=-1  VariantActivationTime=update diagram  Latency=0  AutoFrameSizeCalculation=off
  KuMDFM_DCLinkOVECntDownLimit_NULL : Constant  Value=KuMDFM_DCLinkOVECntDownLimit_NULL
  KuMDFM_DCLinkOVECntDownRate_NULL : Constant  Value=KuMDFM_DCLinkOVECntDownRate_NULL
  KuMDFM_DCLinkOVECntUpLimit_NULL : Constant  Value=KuMDFM_DCLinkOVECntUpLimit_NULL
  KuMDFM_DCLinkOVECntUpRate_NULL : Constant  Value=KuMDFM_DCLinkOVECntUpRate_NULL
  Relational Operator : RelationalOperator  Operator=>  OutDataTypeStr=boolean  InputSameDT=off
  VuMDFM_DCLinkOverVolErrCnt_NULL : Outport
  VbMDFM_DCLinkOverVolErr_flg : Outport  Port=2
  wires:
  Err_Debounce/1 -> Data Type Conversion/1
  Err_Debounce/2 -> VbMDFM_DCLinkOverVolErr_flg/1
  KuMDFM_DCLinkOVECntUpRate_NULL/1 -> Err_Debounce/2
  KuMDFM_DCLinkOVECntUpLimit_NULL/1 -> Err_Debounce/3
  KuMDFM_DCLinkOVECntDownRate_NULL/1 -> Err_Debounce/4
  KuMDFM_DCLinkOVECntDownLimit_NULL/1 -> Err_Debounce/5
  Relational Operator/1 -> Err_Debounce/1
  Constant/1 -> Relational Operator/2
  Data Type Conversion/1 -> VuMDFM_DCLinkOverVolErrCnt_NULL/1  "VuMDFM_DCLinkOverVolErrCnt_NULL"
  VfMDSP_DCLinkVolVal_V/1 -> Relational Operator/1

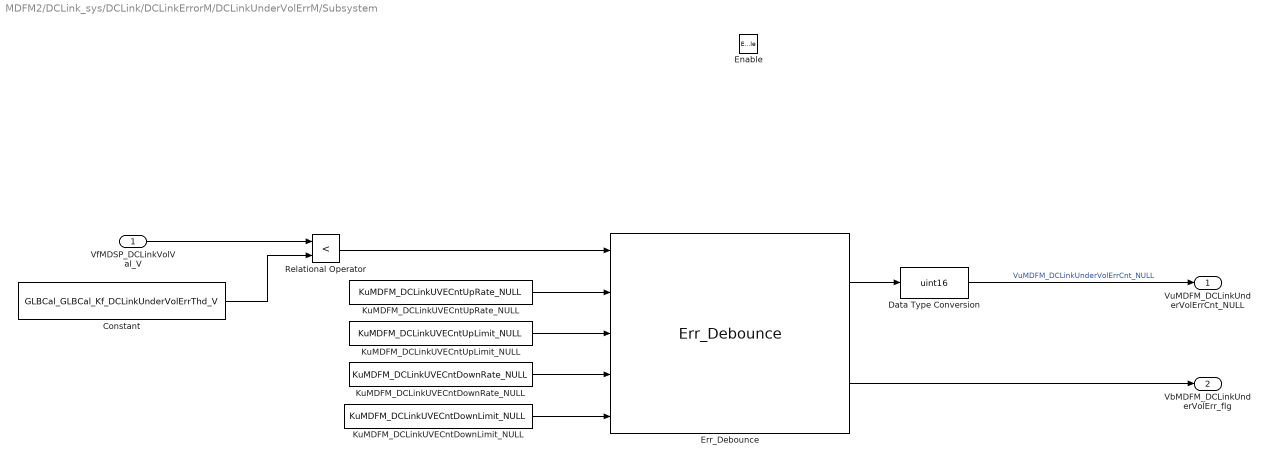
== system MDFM2/DCLink_sys/DCLink/DCLinkErrorM/DCLinkUnderVolErrM/Subsystem ==
  VfMDSP_DCLinkVolVal_V : Inport
  Enable : EnablePort  StatesWhenEnabling=reset
      settings: AttributesFormatString=%<StatesWhenEnabling>
  Constant : Constant  Value=GLBCal_GLBCal_Kf_DCLinkUnderVolErrThd_V
  Data Type Conversion : DataTypeConversion  OutDataTypeStr=uint16  SaturateOnIntegerOverflow=off  RndMeth=Floor
  Err_Debounce : PMSM_Library/Err_Debounce  SystemSampleTime=-1  VariantActivationTime=update diagram  Latency=0  AutoFrameSizeCalculation=off
  KuMDFM_DCLinkUVECntDownLimit_NULL : Constant  Value=KuMDFM_DCLinkUVECntDownLimit_NULL
  KuMDFM_DCLinkUVECntDownRate_NULL : Constant  Value=KuMDFM_DCLinkUVECntDownRate_NULL
  KuMDFM_DCLinkUVECntUpLimit_NULL : Constant  Value=KuMDFM_DCLinkUVECntUpLimit_NULL
  KuMDFM_DCLinkUVECntUpRate_NULL : Constant  Value=KuMDFM_DCLinkUVECntUpRate_NULL
  Relational Operator : RelationalOperator  Operator=<  OutDataTypeStr=boolean  InputSameDT=off
  VuMDFM_DCLinkUnderVolErrCnt_NULL : Outport
  VbMDFM_DCLinkUnderVolErr_flg : Outport  Port=2
  wires:
  KuMDFM_DCLinkUVECntDownLimit_NULL/1 -> Err_Debounce/5
  KuMDFM_DCLinkUVECntDownRate_NULL/1 -> Err_Debounce/4
  KuMDFM_DCLinkUVECntUpLimit_NULL/1 -> Err_Debounce/3
  KuMDFM_DCLinkUVECntUpRate_NULL/1 -> Err_Debounce/2
  Err_Debounce/2 -> VbMDFM_DCLinkUnderVolErr_flg/1
  Err_Debounce/1 -> Data Type Conversion/1
  Constant/1 -> Relational Operator/2
  Relational Operator/1 -> Err_Debounce/1
  Data Type Conversion/1 -> VuMDFM_DCLinkUnderVolErrCnt_NULL/1  "VuMDFM_DCLinkUnderVolErrCnt_NULL"
  VfMDSP_DCLinkVolVal_V/1 -> Relational Operator/1

== system MDFM2/DCLink_sys/DCLink/DCLinkWarnM/DCLinkOverVolWarnM/OverVolReduceCoef ==
  VfMDSP_DCLinkVolVal_V : Inport
  KfMDFM_OverVolPowerOutoutSetPoint_V : Constant  Value=KfMDFM_OverVolPowerOutoutSetPoint_V  OutDataTypeStr=single
  KfMDFM_OverVolPowerOutputFactor_NULL : Constant  Value=KfMDFM_OverVolPowerOutputFactor_NULL  OutDataTypeStr=single
  Lookup Table Dynamic : simulink/Lookup Tables/Lookup Table Dynamic  LookUpMeth=Interpolation-Use End Values  OutDataType=fixdt('single')  OutScaling=[]  OutputDataTypeScalingMode=Specify via dialog  OutDataTypeStr=fixdt('single')  DoSatur=off
  Saturation : Saturate  UpperLimit=1  LowerLimit=0.01
  PowerFactor : Outport
  wires:
  Saturation/1 -> PowerFactor/1
  VfMDSP_DCLinkVolVal_V/1 -> Lookup Table Dynamic/1
  Lookup Table Dynamic/1 -> Saturation/1
  KfMDFM_OverVolPowerOutoutSetPoint_V/1 -> Lookup Table Dynamic/2
  KfMDFM_OverVolPowerOutputFactor_NULL/1 -> Lookup Table Dynamic/3

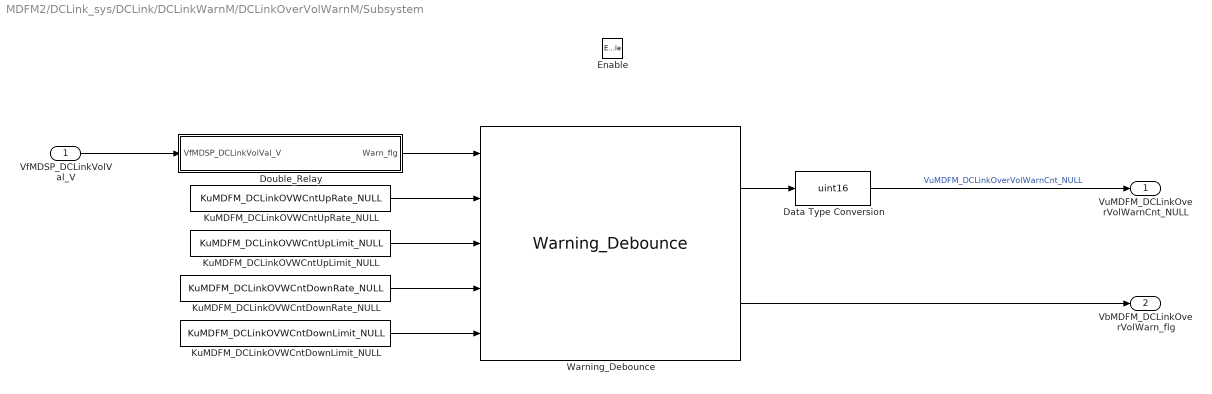
== system MDFM2/DCLink_sys/DCLink/DCLinkWarnM/DCLinkOverVolWarnM/Subsystem ==
  VfMDSP_DCLinkVolVal_V : Inport
  Enable : EnablePort  StatesWhenEnabling=reset
      settings: AttributesFormatString=%<StatesWhenEnabling>
  Data Type Conversion : DataTypeConversion  OutDataTypeStr=uint16  SaturateOnIntegerOverflow=off  RndMeth=Floor
  Double_Relay : Subsystem
  KuMDFM_DCLinkOVWCntDownLimit_NULL : Constant  Value=KuMDFM_DCLinkOVWCntDownLimit_NULL
  KuMDFM_DCLinkOVWCntDownRate_NULL : Constant  Value=KuMDFM_DCLinkOVWCntDownRate_NULL
  KuMDFM_DCLinkOVWCntUpLimit_NULL : Constant  Value=KuMDFM_DCLinkOVWCntUpLimit_NULL
  KuMDFM_DCLinkOVWCntUpRate_NULL : Constant  Value=KuMDFM_DCLinkOVWCntUpRate_NULL
  Warning_Debounce : PMSM_Library/Warning_Debounce  SystemSampleTime=-1  VariantActivationTime=update diagram  Latency=0  AutoFrameSizeCalculation=off
  VuMDFM_DCLinkOverVolWarnCnt_NULL : Outport
  VbMDFM_DCLinkOverVolWarn_flg : Outport  Port=2
  wires:
  Warning_Debounce/1 -> Data Type Conversion/1
  Warning_Debounce/2 -> VbMDFM_DCLinkOverVolWarn_flg/1
  KuMDFM_DCLinkOVWCntUpRate_NULL/1 -> Warning_Debounce/2
  KuMDFM_DCLinkOVWCntUpLimit_NULL/1 -> Warning_Debounce/3
  KuMDFM_DCLinkOVWCntDownRate_NULL/1 -> Warning_Debounce/4
  KuMDFM_DCLinkOVWCntDownLimit_NULL/1 -> Warning_Debounce/5
  Double_Relay/1(Warn_flg) -> Warning_Debounce/1
  Data Type Conversion/1 -> VuMDFM_DCLinkOverVolWarnCnt_NULL/1  "VuMDFM_DCLinkOverVolWarnCnt_NULL"
  VfMDSP_DCLinkVolVal_V/1 -> Double_Relay/1(VfMDSP_DCLinkVolVal_V)

== system MDFM2/DCLink_sys/DCLink/DCLinkWarnM/DCLinkUnderVolWarnM/Subsystem ==
  note: % U nder V oltage W arning
  VfMDSP_DCLinkVolVal_V : Inport
  Enable : EnablePort  StatesWhenEnabling=reset
      settings: AttributesFormatString=%<StatesWhenEnabling>
  Data Type Conversion : DataTypeConversion  OutDataTypeStr=uint16  SaturateOnIntegerOverflow=off  RndMeth=Floor
  Double_Relay : Subsystem
  KuMDFM_DCLinkUVWCntDownLimit_NULL : Constant  Value=KuMDFM_DCLinkUVWCntDownLimit_NULL
  KuMDFM_DCLinkUVWCntDownRate_NULL : Constant  Value=KuMDFM_DCLinkUVWCntDownRate_NULL
  KuMDFM_DCLinkUVWCntUpLimit_NULL : Constant  Value=KuMDFM_DCLinkUVWCntUpLimit_NULL
  KuMDFM_DCLinkUVWCntUpRate_NULL : Constant  Value=KuMDFM_DCLinkUVWCntUpRate_NULL
  Warning_Debounce : PMSM_Library/Warning_Debounce  SystemSampleTime=-1  VariantActivationTime=update diagram  Latency=0  AutoFrameSizeCalculation=off
  VuMDFM_DCLinkUnderVolWarnCnt_NULL : Outport
  VbMDFM_DCLinkUnderVolWarn_flg : Outport  Port=2
  wires:
  KuMDFM_DCLinkUVWCntDownLimit_NULL/1 -> Warning_Debounce/5
  KuMDFM_DCLinkUVWCntDownRate_NULL/1 -> Warning_Debounce/4
  KuMDFM_DCLinkUVWCntUpLimit_NULL/1 -> Warning_Debounce/3
  KuMDFM_DCLinkUVWCntUpRate_NULL/1 -> Warning_Debounce/2
  Warning_Debounce/2 -> VbMDFM_DCLinkUnderVolWarn_flg/1
  Warning_Debounce/1 -> Data Type Conversion/1
  Double_Relay/1(Warn_flg) -> Warning_Debounce/1
  Data Type Conversion/1 -> VuMDFM_DCLinkUnderVolWarnCnt_NULL/1  "VuMDFM_DCLinkUnderVolWarnCnt_NULL"
  VfMDSP_DCLinkVolVal_V/1 -> Double_Relay/1(VfMDSP_DCLinkVolVal_V)

== system MDFM2/DCLink_sys/DCLink/DCLinkWarnM/DCLinkUnderVolWarnM/UnderVolReduceCoef ==
  VfMDSP_DCLinkVolVal_V : Inport
  KfMDFM_UnderVolPowerOutoutSetPoint_V : Constant  Value=KfMDFM_UnderVolPowerOutoutSetPoint_V  OutDataTypeStr=single
  KfMDFM_UnderVolPowerOutputFactor_NULL : Constant  Value=KfMDFM_UnderVolPowerOutputFactor_NULL  OutDataTypeStr=single
  Lookup Table Dynamic : simulink/Lookup Tables/Lookup Table Dynamic  LookUpMeth=Interpolation-Use End Values  OutDataType=fixdt('single')  OutScaling=[]  OutputDataTypeScalingMode=Specify via dialog  OutDataTypeStr=fixdt('single')  DoSatur=off
  Saturation : Saturate  UpperLimit=1  LowerLimit=0.01
  PowerFactor : Outport
  wires:
  Saturation/1 -> PowerFactor/1
  VfMDSP_DCLinkVolVal_V/1 -> Lookup Table Dynamic/1
  Lookup Table Dynamic/1 -> Saturation/1
  KfMDFM_UnderVolPowerOutoutSetPoint_V/1 -> Lookup Table Dynamic/2
  KfMDFM_UnderVolPowerOutputFactor_NULL/1 -> Lookup Table Dynamic/3

== system MDFM2/DCLink_sys/DCLink/DCLinkWarnM/DCLinkOverVolWarnM/Subsystem/Double_Relay ==
  VfMDSP_DCLinkVolVal_V : Inport
  ChkIfWarnWithDoubleThd : PMSM_Library/ChkIfWarnWithDoubleThd  SystemSampleTime=-1  VariantActivationTime=update diagram  Latency=0  AutoFrameSizeCalculation=off
  Constant : Constant  Value=KfMDFM_DCLinkOverVolWarnThd_V
  Constant2 : Constant  Value=GLBCal_GLBCal_Kf_DCLinkOverVolErrThd_V
  Warn_flg : Outport
  wires:
  Constant/1 -> ChkIfWarnWithDoubleThd/3
  Constant2/1 -> ChkIfWarnWithDoubleThd/1
  ChkIfWarnWithDoubleThd/1 -> Warn_flg/1
  VfMDSP_DCLinkVolVal_V/1 -> ChkIfWarnWithDoubleThd/2

== system MDFM2/DCLink_sys/DCLink/DCLinkWarnM/DCLinkUnderVolWarnM/Subsystem/Double_Relay ==
  VfMDSP_DCLinkVolVal_V : Inport
  GLBCal_GLBCal_Kf_DCLinkUnderVolErrThd_V : Constant  Value=GLBCal_GLBCal_Kf_DCLinkUnderVolErrThd_V
  KfMDFM_DCLinkUnderVolWarnThd_V : Constant  Value=KfMDFM_DCLinkUnderVolWarnThd_V
  Logical Operator : Logic  AllPortsSameDT=off  OutDataTypeStr=boolean
  Relational Operator : RelationalOperator  Operator=<  OutDataTypeStr=boolean  InputSameDT=off
  Relational Operator1 : RelationalOperator  Operator=<  OutDataTypeStr=boolean  InputSameDT=off
  Warn_flg : Outport
  wires:
  VfMDSP_DCLinkVolVal_V/1 -> Relational Operator1/2, Relational Operator/1
  GLBCal_GLBCal_Kf_DCLinkUnderVolErrThd_V/1 -> Relational Operator1/1
  KfMDFM_DCLinkUnderVolWarnThd_V/1 -> Relational Operator/2
  Relational Operator/1 -> Logical Operator/2
  Relational Operator1/1 -> Logical Operator/1
  Logical Operator/1 -> Warn_flg/1
